simulink model "ARDroneHoverWin"  (R2014a)
settings: Solver=ode1  StartTime=0.0  StopTime=inf  FixedStep=sampleTime  RelTol=1e-3
values from neighbouring files (symbols this model uses):
  sampleTime = 0.04    [start.m]
undefined symbols (not defined in the file or in its folder): Standard_Devices, UDP_Protocol
libraries: ARBlocks x2, rtwinlib x1
CloseFcn:
  | rtwprivate ssgencode ModelCloseRequest Good_NL_model
settings Model: SimulationMode=external  ExtModeTrigDuration=100000  Creator=Paul  LastModifiedBy=Django
settings DataIOCC: SignalLoggingSaveFormat=ModelDataLogs  TimeSaveName=time
settings OptimizationCC: ExpressionDepthLimit=2147483647  InitFltsAndDblsToZero=on
settings DebuggingCC: UnderspecifiedInitializationDetection=Classic  FcnCallInpInsideContextMsg=UseLocalSettings  StateNameClashWarn=warning
settings HardwareCC: ProdIntDivRoundTo=Zero  ProdEndianess=LittleEndian  ProdHWDeviceType=Generic->32-bit x86 compatible
settings RTWCC: SystemTargetFile=rtwin.tlc  TemplateMakefile=rtwin.tmf  Description=Real-Time Windows Target  ProcessScript=rtwin_make_rtw_hook  RTWCompilerOptimization=On
settings CodeAppCC: MaxIdLength=95
settings RTWinTargetCC: TargetLibSuffix=_rtwin.lib  TargetPreCompLibLocation=E:\Installationposition\InstallPath\MATLAB\MATLAB2014a\toolbox\rtw\targets\rtwin\lib\win64

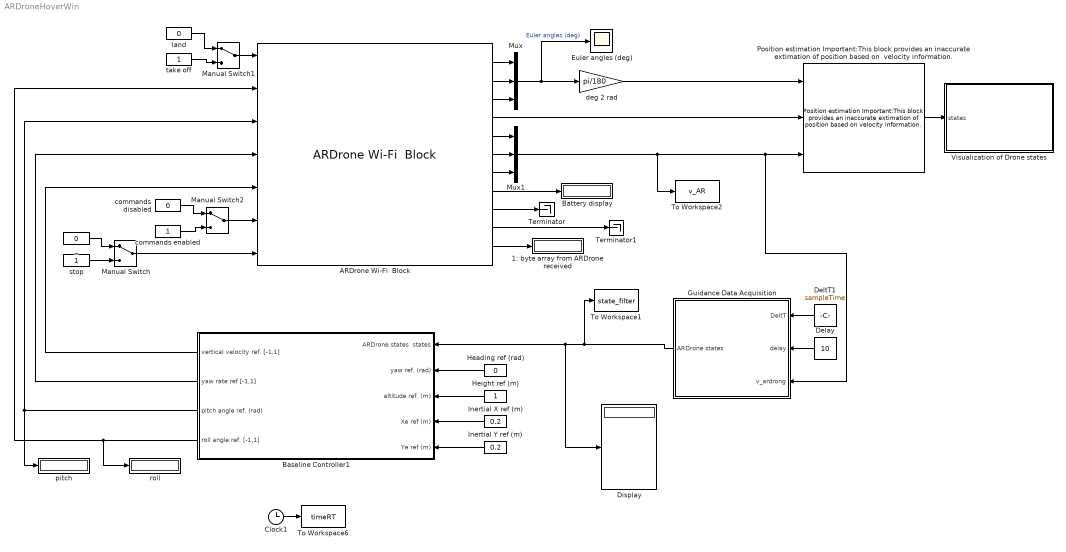
== system ARDroneHoverWin ==
  "1: byte array from ARDrone received " : Display
  ARDrone Wi-Fi  Block : ARBlocks/ARDrone Wi-Fi  Block
  Baseline Controller1 : Subsystem  AncestorBlock=ARBlocks/Baseline Controller
  Battery display : Display
  Clock1 : Clock
  Delay : Constant  Value=10
  DeltT1 : Constant  Value=sampleTime
  Display : Display
  Euler angles (deg) : Scope
      settings: YMin=-10  YMax=120  MaxDataPoints=500000
  Guidance Data Acquisition : Subsystem  AncestorBlock=ARBlocks/Guidance Data Acquisition
  Heading ref (rad) : Constant  Value=0
  Height ref (m) : Constant
  Inertial X ref (m) : Constant  Value=0.2
  Inertial Y ref (m) : Constant  Value=0.2
  Manual Switch : ManualSwitch
  Manual Switch1 : ManualSwitch
  Manual Switch2 : ManualSwitch
  Mux : Mux  Inputs=3
  Mux1 : Mux  Inputs=3
  "Position estimation Important:This block provides an inaccurate extimation of position based on  velocity information. " : ARBlocks/Position estimation Important:This block provides an  inaccurate extimation of position  based on  velocity information. 
  Terminator : Terminator
  Terminator1 : Terminator
  To Workspace1 : ToWorkspace  VariableName=state_filter  SampleTime=-1
  To Workspace2 : ToWorkspace  VariableName=v_AR  SampleTime=-1
  To Workspace6 : ToWorkspace  VariableName=timeRT  SampleTime=sampleTime
  Visualization of Drone states : Subsystem
  _ : Constant  Value=0
  commands disabled : Constant  Value=0
  commands enabled : Constant
  deg 2 rad : Gain  Gain=pi/180
  land : Constant  Value=0
  pitch : Display
  roll : Display
  stop : Constant
  take off : Constant
  wires:
  _/1 -> Manual Switch/1
  stop/1 -> Manual Switch/2
  land/1 -> Manual Switch1/1
  take off/1 -> Manual Switch1/2
  commands disabled/1 -> Manual Switch2/1
  commands enabled/1 -> Manual Switch2/2
  Manual Switch1/1 -> ARDrone Wi-Fi  Block/1
  Manual Switch2/1 -> ARDrone Wi-Fi  Block/6
  Manual Switch/1 -> ARDrone Wi-Fi  Block/7
  ARDrone Wi-Fi  Block/1 -> Mux/1
  ARDrone Wi-Fi  Block/2 -> Mux/2
  ARDrone Wi-Fi  Block/5 -> Mux1/1
  ARDrone Wi-Fi  Block/6 -> Mux1/2
  ARDrone Wi-Fi  Block/7 -> Mux1/3
  Mux/1 -> Euler angles (deg)/1, deg 2 rad/1  "Euler angles (deg)"
  ARDrone Wi-Fi  Block/8 -> Battery display/1
  Baseline Controller1/1(vertical velocity ref. [-1,1]) -> ARDrone Wi-Fi  Block/5
  Baseline Controller1/3(pitch angle ref. (rad)) -> pitch/1, ARDrone Wi-Fi  Block/3
  "Position estimation Important:This block provides an inaccurate extimation of position based on  velocity information. "/1 -> Visualization of Drone states/1(states)
  deg 2 rad/1 -> "Position estimation Important:This block provides an inaccurate extimation of position based on  velocity information. "/1
  ARDrone Wi-Fi  Block/4 -> "Position estimation Important:This block provides an inaccurate extimation of position based on  velocity information. "/2
  Baseline Controller1/4(roll angle ref. [-1,1]) -> roll/1, ARDrone Wi-Fi  Block/2
  ARDrone Wi-Fi  Block/3 -> Mux/3
  ARDrone Wi-Fi  Block/9 -> Terminator/1
  ARDrone Wi-Fi  Block/10 -> Terminator1/1
  ARDrone Wi-Fi  Block/11 -> "1: byte array from ARDrone received "/1
  Baseline Controller1/2(yaw rate ref [-1,1]) -> ARDrone Wi-Fi  Block/4
  Clock1/1 -> To Workspace6/1
  Height ref (m)/1 -> Baseline Controller1/3(altitude ref. (m))
  Inertial X ref (m)/1 -> Baseline Controller1/4(Xe ref (m))
  Inertial Y ref (m)/1 -> Baseline Controller1/5(Ye ref (m))
  Heading ref (rad)/1 -> Baseline Controller1/2(yaw ref. (rad))
  Guidance Data Acquisition/1(ARDrone states) -> To Workspace1/1, Display/1, Baseline Controller1/1("ARDrone states  states ")
  DeltT1/1 -> Guidance Data Acquisition/1(DeltT)
  Mux1/1 -> To Workspace2/1, Guidance Data Acquisition/3(v_ardrong), "Position estimation Important:This block provides an inaccurate extimation of position based on  velocity information. "/3
  Delay/1 -> Guidance Data Acquisition/2(delay)

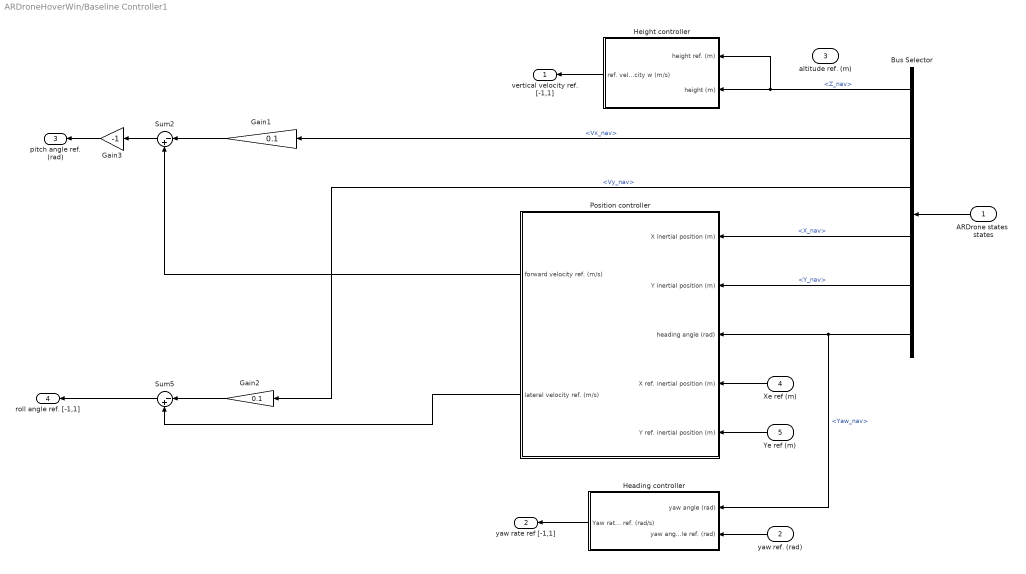
== system ARDroneHoverWin/Baseline Controller1 ==
  "ARDrone states  states " : Inport
  yaw ref. (rad) : Inport  Port=2
  altitude ref. (m) : Inport  Port=3
  Xe ref (m) : Inport  Port=4
  Ye ref (m) : Inport  Port=5
  Bus Selector : BusSelector  OutputSignals=Z_nav,Vx_nav,Vy_nav,X_nav,Y_nav,Yaw_nav
  Gain1 : Gain  Gain=0.1
  Gain2 : Gain  Gain=0.1
  Gain3 : Gain  Gain=-1
  Heading controller : Subsystem
  "Height controller " : Subsystem
  Position controller : Subsystem
  Sum2 : Sum  Inputs=|-+
  Sum5 : Sum  Inputs=|-+
  vertical velocity ref. [-1,1] : Outport
  yaw rate ref [-1,1] : Outport  Port=2
  pitch angle ref. (rad) : Outport  Port=3
  roll angle ref. [-1,1] : Outport  Port=4
  wires:
  Ye ref (m)/1 -> Position controller/5(Y ref. inertial position (m))
  Xe ref (m)/1 -> Position controller/4(X ref. inertial position (m))
  Bus Selector/5 -> Position controller/2(Y inertial position (m))  "<Y_nav>"
  Bus Selector/4 -> Position controller/1(X inertial position (m))  "<X_nav>"
  Heading controller/1(Yaw rate ref. (rad/s)) -> yaw rate ref [-1,1]/1
  Bus Selector/2 -> Gain1/1  "<Vx_nav>"
  Sum5/1 -> roll angle ref. [-1,1]/1
  "Height controller "/1(ref. velocity w (m/s)) -> vertical velocity ref. [-1,1]/1
  Bus Selector/1 -> "Height controller "/1(height ref. (m)), "Height controller "/2(height (m))  "<Z_nav>"
  "ARDrone states  states "/1 -> Bus Selector/1
  Bus Selector/6 -> Position controller/3(heading angle (rad)), Heading controller/1(yaw angle (rad))  "<Yaw_nav>"
  Sum2/1 -> Gain3/1
  Gain1/1 -> Sum2/1
  Gain3/1 -> pitch angle ref. (rad)/1
  Position controller/1(forward velocity ref. (m/s)) -> Sum2/2
  Gain2/1 -> Sum5/1
  Position controller/2(lateral velocity ref. (m/s)) -> Sum5/2
  Bus Selector/3 -> Gain2/1  "<Vy_nav>"
  yaw ref. (rad)/1 -> Heading controller/2(yaw angle ref. (rad))

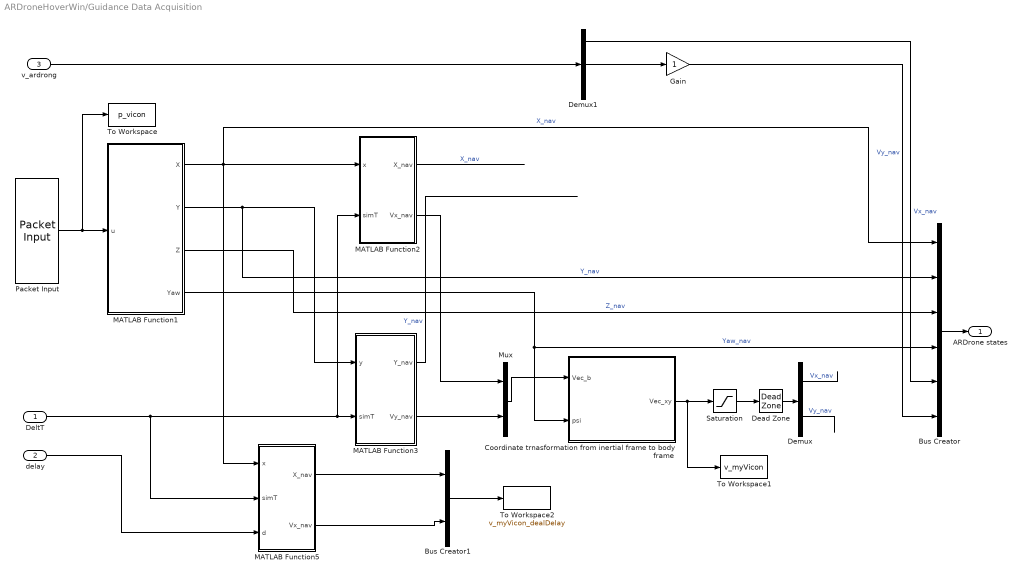
== system ARDroneHoverWin/Guidance Data Acquisition ==
  DeltT : Inport
  delay : Inport  Port=2
  v_ardrong : Inport  Port=3
  Bus Creator : BusCreator  Inputs=6
  Bus Creator1 : BusCreator  Inputs=2
  "Coordinate trnasformation from inertial frame to body frame " : MATLAB Function  TreatAsAtomicUnit=on
  Dead Zone : DeadZone  LowerValue=-0.005  UpperValue=0.005  SaturateOnIntegerOverflow=on
  Demux : Demux  Outputs=2
  Demux1 : Demux  Outputs=3
  Gain : Gain
  MATLAB Function1 : MATLAB Function  TreatAsAtomicUnit=on
  MATLAB Function2 : MATLAB Function  TreatAsAtomicUnit=on
  MATLAB Function3 : MATLAB Function  TreatAsAtomicUnit=on
  MATLAB Function5 : MATLAB Function  TreatAsAtomicUnit=on
  Mux : Mux  Inputs=2
  Packet Input : rtwinlib/Packet Input  SampleTime=sampleTime  MaxMissedTicks=1  ShowMissedTicks=off  YieldWhenWaiting=on  DrvName=Standard_Devices/UDP_Protocol  DrvAddress=5500  DrvOptions=[3215458314 5502]  PacketSize=48  DataTypes='6*double'  ShowReady=off  ShowError=off  PacketID=1  ByteOrder=2  ShowTimestamp=off
      settings: AttributesFormatString=Standard Devices\nUDP Protocol [157Ch]
  Saturation : Saturate  UpperLimit=1  LowerLimit=-1
  To Workspace : ToWorkspace  VariableName=p_vicon  SampleTime=-1
  To Workspace1 : ToWorkspace  VariableName=v_myVicon  SampleTime=-1
  To Workspace2 : ToWorkspace  VariableName=v_myVicon_dealDelay  SampleTime=-1
  ARDrone states : Outport
  wires:
  Bus Creator/1 -> ARDrone states/1
  MATLAB Function1/4(Yaw) -> Bus Creator/4, "Coordinate trnasformation from inertial frame to body frame "/2(psi)  "Yaw_nav"
  MATLAB Function1/3(Z) -> Bus Creator/3  "Z_nav"
  Packet Input/1 -> To Workspace/1, MATLAB Function1/1(u)
  Mux/1 -> "Coordinate trnasformation from inertial frame to body frame "/1(Vec_b)
  Demux/1 -> ?  "Vx_nav"
  Demux/2 -> ?  "Vy_nav"
  Dead Zone/1 -> Demux/1
  "Coordinate trnasformation from inertial frame to body frame "/1(Vec_xy) -> Saturation/1, To Workspace1/1
  Saturation/1 -> Dead Zone/1
  MATLAB Function3/2(Vy_nav) -> Mux/2
  MATLAB Function2/2(Vx_nav) -> Mux/1
  MATLAB Function2/1(X_nav) -> ?  "X_nav"
  MATLAB Function3/1(Y_nav) -> ?  "Y_nav"
  MATLAB Function1/1(X) -> Bus Creator/1, MATLAB Function5/1(x), MATLAB Function2/1(x)  "X_nav"
  DeltT/1 -> MATLAB Function5/2(simT), MATLAB Function2/2(simT), MATLAB Function3/2(simT)
  delay/1 -> MATLAB Function5/3(d)
  MATLAB Function5/1(X_nav) -> Bus Creator1/1
  MATLAB Function5/2(Vx_nav) -> Bus Creator1/2
  Bus Creator1/1 -> To Workspace2/1
  MATLAB Function1/2(Y) -> MATLAB Function3/1(y), Bus Creator/2  "Y_nav"
  v_ardrong/1 -> Demux1/1
  Demux1/1 -> Bus Creator/5  "Vx_nav"
  Demux1/2 -> Gain/1
  Gain/1 -> Bus Creator/6  "Vy_nav"

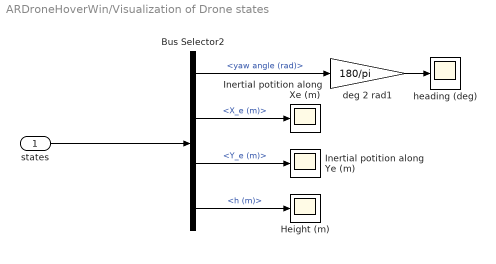
== system ARDroneHoverWin/Visualization of Drone states ==
  states : Inport
  Bus Selector2 : BusSelector  OutputSignals=yaw angle (rad),X_e (m),Y_e (m),h (m)
  Height (m) : Scope
      settings: YMin=-22.5  YMax=22.5  SaveName=ScopeData5  MaxDataPoints=500000
  Inertial potition along Xe (m) : Scope
      settings: YMin=-22.5  YMax=22.5  SaveName=ScopeData3  MaxDataPoints=500000
  Inertial potition along Ye (m) : Scope
      settings: YMin=-22.5  YMax=22.5  SaveName=ScopeData4  MaxDataPoints=500000
  deg 2 rad1 : Gain  Gain=180/pi
  heading (deg) : Scope
      settings: YMin=-22.5  YMax=22.5  SaveName=ScopeData2  MaxDataPoints=500000
  wires:
  states/1 -> Bus Selector2/1
  Bus Selector2/1 -> deg 2 rad1/1  "<yaw angle (rad)>"
  Bus Selector2/2 -> Inertial potition along Xe (m)/1  "<X_e (m)>"
  Bus Selector2/3 -> Inertial potition along Ye (m)/1  "<Y_e (m)>"
  Bus Selector2/4 -> Height (m)/1  "<h (m)>"
  deg 2 rad1/1 -> heading (deg)/1

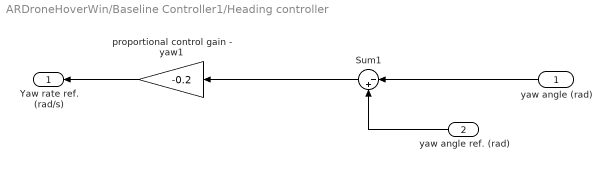
== system ARDroneHoverWin/Baseline Controller1/Heading controller ==
  yaw angle (rad) : Inport
  yaw angle ref. (rad) : Inport  Port=2
  Sum1 : Sum  Inputs=|-+
  proportional control gain - yaw1 : Gain  Gain=-0.2
  Yaw rate ref. (rad/s) : Outport
  wires:
  yaw angle ref. (rad)/1 -> Sum1/2
  yaw angle (rad)/1 -> Sum1/1
  proportional control gain - yaw1/1 -> Yaw rate ref. (rad/s)/1
  Sum1/1 -> proportional control gain - yaw1/1

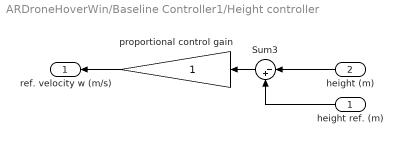
== system ARDroneHoverWin/Baseline Controller1/Height controller  ==
  height ref. (m) : Inport
  height (m) : Inport  Port=2
  Sum3 : Sum  Inputs=|-+
  proportional control gain : Gain
  ref. velocity w (m/s) : Outport
  wires:
  height ref. (m)/1 -> Sum3/2
  height (m)/1 -> Sum3/1
  Sum3/1 -> proportional control gain/1
  proportional control gain/1 -> ref. velocity w (m/s)/1

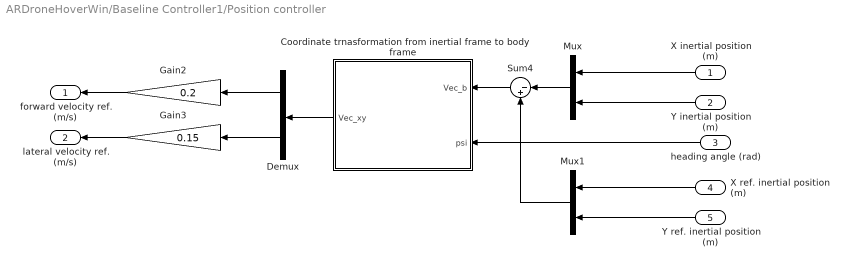
== system ARDroneHoverWin/Baseline Controller1/Position controller ==
  X inertial position (m) : Inport
  Y inertial position (m) : Inport  Port=2
  heading angle (rad) : Inport  Port=3
  X ref. inertial position (m) : Inport  Port=4
  Y ref. inertial position (m) : Inport  Port=5
  "Coordinate trnasformation from inertial frame to body frame " : MATLAB Function  TreatAsAtomicUnit=on
  Demux : Demux  Outputs=2
  Gain2 : Gain  Gain=0.2
  Gain3 : Gain  Gain=0.15
  Mux : Mux  Inputs=2
  Mux1 : Mux  Inputs=2
  Sum4 : Sum  Inputs=|-+
  forward velocity ref. (m/s) : Outport
  lateral velocity ref. (m/s) : Outport  Port=2
  wires:
  Gain3/1 -> lateral velocity ref. (m/s)/1
  Demux/2 -> Gain3/1
  Demux/1 -> Gain2/1
  Y ref. inertial position (m)/1 -> Mux1/2
  X ref. inertial position (m)/1 -> Mux1/1
  Mux/1 -> Sum4/1
  X inertial position (m)/1 -> Mux/1
  Y inertial position (m)/1 -> Mux/2
  Sum4/1 -> "Coordinate trnasformation from inertial frame to body frame "/1(Vec_b)
  Mux1/1 -> Sum4/2
  "Coordinate trnasformation from inertial frame to body frame "/1(Vec_xy) -> Demux/1
  heading angle (rad)/1 -> "Coordinate trnasformation from inertial frame to body frame "/2(psi)
  Gain2/1 -> forward velocity ref. (m/s)/1

== matlab function ARDroneHoverWin/Guidance Data Acquisition/Coordinate trnasformation from inertial frame to body frame  ==
  data: Vec_b input; Vec_xy output; psi input
function Vec_xy  = fcn(Vec_b , psi)
%#codegen
T = [cos(psi) sin(psi) ; sin(psi) -cos(psi)] ; 
Vec_xy = T*Vec_b(1:2,1);

== matlab function ARDroneHoverWin/Guidance Data Acquisition/MATLAB Function1 ==
  data: X output; u input; Y output; Z output; Yaw output
function [X,Y,Z,Yaw] = fcn(u)
X = u(1)/1000;
Y = u(2)/1000;
Z = u(3)/1000;
Yaw = u(5);
end

== matlab function ARDroneHoverWin/Guidance Data Acquisition/MATLAB Function2 ==
  data: x input; X_nav output; Vx_nav output; simT input
function [X_nav,Vx_nav] = fcn(x,simT)
persistent Phi;
if isempty(Phi)
    Phi = [1 simT;0 1];
end

persistent Tao;
if isempty(Tao)
    Tao = [0 simT]';
end

persistent Q;
if isempty(Q)
    Q = 50;
end

persistent H;
if isempty(H)
    H = [1 0];
end

persistent R;
if isempty(R)
    R = 7.81e-1;
end

persistent Xe;
if isempty(Xe)
    Xe = [0 0]';
end

persistent X_e;
if isempty(X_e)
    X_e = [0 0]';
end

persistent Z_e;
if isempty(Z_e)
    Z_e = 0;
end

persistent P;
if isempty(P)
    P = Q*[1 0;0 1]; % 估计误差协方差阵
end

persistent P_;
if isempty(P_)
    P_ = Q*[1 0;0 1]; % 估计误差协方差阵
end

% 状态变量的先验估计
X_e = Phi*Xe;
% 观测向量的先验估计
Z_e = H*X_e;
% 计算先验估计误差协方差阵
P_ = Phi*P*Phi'+Tao*Q*Tao';

% 观测值 [x y z yaw]'  输入Z=[x y z pitch yaw roll vx vy vz]'
Zm = x;

% 计算卡尔曼增益
Kk = P_*H'*(inv(H*P_*H'+R));
% 计算后验估计
Xe = X_e+Kk*(Zm-Z_e);
% 计算后验协方差阵
P=(eye(2)-Kk*H)*P_;

X_nav = Xe(1);
Vx_nav = Xe(2);
end

== matlab function ARDroneHoverWin/Guidance Data Acquisition/MATLAB Function3 ==
  data: y input; Y_nav output; Vy_nav output; simT input
function [Y_nav,Vy_nav] = fcn(y,simT)
persistent Phi;
if isempty(Phi)
    Phi = [1 simT;0 1];
end

persistent Tao;
if isempty(Tao)
    Tao = [0 simT]';
end

persistent Q;
if isempty(Q)
    Q = 50;
end

persistent H;
if isempty(H)
    H = [1 0];
end

persistent R;
if isempty(R)
    R = 2.33e-1;
end

persistent Xe;
if isempty(Xe)
    Xe = [0 0]';
end

persistent X_e;
if isempty(X_e)
    X_e = [0 0]';
end

persistent Z_e;
if isempty(Z_e)
    Z_e = 0;
end

persistent P;
if isempty(P)
    P = Q*[1 0;0 1]; % 估计误差协方差阵
end

persistent P_;
if isempty(P_)
    P_ = Q*[1 0;0 1]; % 估计误差协方差阵
end

% 状态变量的先验估计
X_e = Phi*Xe;
% 观测向量的先验估计
Z_e = H*X_e;
% 计算先验估计误差协方差阵
P_ = Phi*P*Phi'+Tao*Q*Tao';

% 观测值 [x y z yaw]'  输入Z=[x y z pitch yaw roll vx vy vz]'
Zm = y;

% 计算卡尔曼增益
Kk = P_*H'*(inv(H*P_*H'+R));
% 计算后验估计
Xe = X_e+Kk*(Zm-Z_e);
% 计算后验协方差阵
P=(eye(2)-Kk*H)*P_;

Y_nav = Xe(1);
Vy_nav = Xe(2);
end

== matlab function ARDroneHoverWin/Guidance Data Acquisition/MATLAB Function5 ==
  data: x input; X_nav output; Vx_nav output; simT input; d input
function [X_nav,Vx_nav] = fcn(x,simT,d)
persistent Phi;
if isempty(Phi)
    Phi = [1 simT;0 1];
end

persistent Tao;
if isempty(Tao)
    Tao = [0 simT]';
end

persistent Q;
if isempty(Q)
    Q = 50;
end

persistent H;
if isempty(H)
    H = [1 0];
end

persistent R;
if isempty(R)
    R = 7.81e-1;
end

persistent Xe;
if isempty(Xe)
    Xe = [0 0]';
end

persistent X_e;
if isempty(X_e)
    X_e = zeros(2,10);
end

persistent Z_e;
if isempty(Z_e)
    Z_e = zeros(10);
end

persistent P;
if isempty(P)
    P = Q*[1 0;0 1]; % 估计误差协方差阵
end

persistent P_;
if isempty(P_)
    P_ = zeros(2,2,10);
    for i=1:10
        P_(:,:,i) = P;  % 估计误差协方差阵
    end 
end

% 状态变量的先验估计
X_e(:,d) = Phi*Xe;
% 观测向量的先验估计
Z_e(:,d) = H*X_e(:,d);
% 计算先验估计误差协方差阵
P_(:,:,d) = Phi*P*Phi'+Tao*Q*Tao';

% 观测值x
Zm = x;

% 计算卡尔曼增益
Kk = P_(:,:,1)*H'*(inv(H*P_(:,:,1)*H'+R));
% 计算后验估计
Xe = X_e(:,1)+Kk*(Zm-Z_e(1));
% 计算后验协方差阵
P=(eye(2)-Kk*H)*P_(:,:,1);

% 更新缓冲区
X_e(:,1:d-1) = X_e(:,2:d);
Z_e(:,1:d-1) = Z_e(:,2:d);
P_(:,:,1:d-1) = P_(:,:,2:d);

% 往前预测直到当前时刻
for i=1:d
    Xe = Phi*Xe; 
end
X_nav = Xe(1);
Vx_nav = Xe(2);

% persistent Phi;
% if isempty(Phi)
%     Phi = [1 simT;0 1];
% end
% 
% persistent Tao;
% if isempty(Tao)
%     Tao = [0 simT]';
% end
% 
% persistent Q;
% if isempty(Q)
%     Q = 50;
% end
% 
% persistent H;
% if isempty(H)
%     H = [1 0];
% end
% 
% persistent R;
% if isempty(R)
%     R = 7.81e-1;
% end
% 
% persistent Xe;
% if isempty(Xe)
%     Xe = [0 0]';
% end
% 
% persistent X_e;
% if isempty(X_e)
%     X_e = [0 0]';
% end
% 
% persistent Z_e;
% if isempty(Z_e)
%     Z_e = 0;
% end
% 
% persistent P;
% if isempty(P)
%     P = Q*[1 0;0 1]; % 估计误差协方差阵
% end
% 
% persistent P_;
% if isempty(P_)
%     P_ = Q*[1 0;0 1]; % 估计误差协方差阵
% end
% 
% % 状态变量的先验估计
% X_e = Phi*Xe;
% % 观测向量的先验估计
% Z_e = H*X_e;
% % 计算先验估计误差协方差阵
% P_ = Phi*P*Phi'+Tao*Q*Tao';
% 
% % 观测值 [x y z yaw]'  输入Z=[x y z pitch yaw roll vx vy vz]'
% Zm = x;
% 
% % 计算卡尔曼增益
% Kk = P_*H'*(inv(H*P_*H'+R));
% % 计算后验估计
% Xe = X_e+Kk*(Zm-Z_e);
% % 计算后验协方差阵
% P=(eye(2)-Kk*H)*P_;
% 
% X_nav = Xe(1);
% Vx_nav = Xe(2);
end

== matlab function ARDroneHoverWin/Baseline Controller1/Position controller/Coordinate trnasformation from inertial frame to body frame  ==
  data: Vec_b input; Vec_xy output; psi input
function Vec_xy  = fcn(Vec_b , psi)
%#codegen
T = [cos(psi) sin(psi) ; sin(psi) -cos(psi)] ; 
Vec_xy = T*Vec_b(1:2,1);
